simulink model "SOGI_test"  (R2016a)
settings: Solver=VariableStepAuto  StartTime=0.0  StopTime=1  RelTol=1e-3
libraries: powerlib x3, powerlib_meascontrol x2, simulink x1
settings Model: Creator=13641  LastModifiedBy=HDM

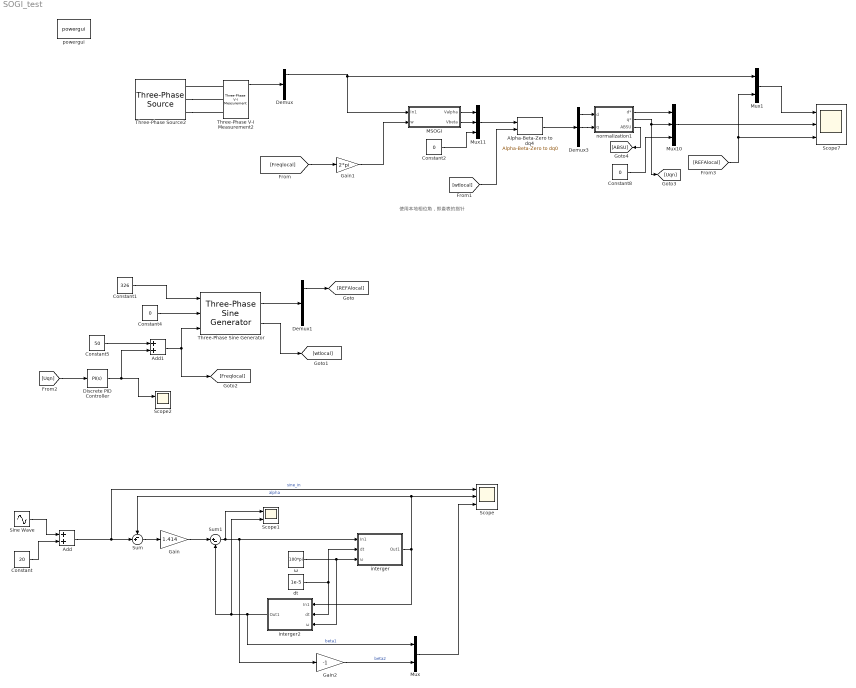
== system SOGI_test ==
  note: 使用本地相位角，即查表的指针
  Add : Sum
  Add1 : Sum
  Alpha-Beta-Zero to dq4 : powerlib_meascontrol/Transformations/Alpha-Beta-Zero to dq0  Alignment=90 degrees behind phase A axis
  Constant : Constant  Value=20
  Constant1 : Constant  Value=326
  Constant2 : Constant  Value=0
  Constant4 : Constant  Value=0
  Constant5 : Constant  Value=50
  Constant8 : Constant  Value=0
  Demux : Demux  Outputs=3
  Demux1 : Demux  Outputs=3
  Demux3 : Demux  Outputs=3
  Discrete PID Controller : simulink/Continuous/PID Controller  Controller=PI  TimeDomain=Continuous-time  SampleTime=-1  IntegratorMethod=Forward Euler  FilterMethod=Forward Euler  Form=Parallel  UseFilter=on  ControllerParametersSource=internal  P=5  I=20  D=0  N=100  InitialConditionSource=internal  InitialConditionForIntegrator=0  InitialConditionForFilter=0  ExternalReset=none  LimitOutput=off  UpperSaturationLimit=inf  LowerSaturationLimit=-inf  LinearizeAsGain=off  AntiWindupMode=none  Kb=1  TrackingMode=off  Kt=1  PParamMin=[]  PParamMax=[]  IParamMin=[]  IParamMax=[]  DParamMin=[]  DParamMax=[]  NParamMin=[]  NParamMax=[]  KbParamMin=[]  KbParamMax=[]  KtParamMin=[]  KtParamMax=[]  POutMin=[]  POutMax=[]  IOutMin=[]  IOutMax=[]  DOutMin=[]  DOutMax=[]  NOutMin=[]  NOutMax=[]  KbOutMin=[]  KbOutMax=[]  KtOutMin=[]  KtOutMax=[]  IntegratorOutMin=[]  IntegratorOutMax=[]  FilterOutMin=[]  FilterOutMax=[]  SumOutMin=[]  SumOutMax=[]  SumI1OutMin=[]  SumI1OutMax=[]  SumI2OutMin=[]  SumI2OutMax=[]  SumI3OutMin=[]  SumI3OutMax=[]  SumDOutMin=[]  SumDOutMax=[]  SaturationOutMin=[]  SaturationOutMax=[]  IntegratorContinuousStateAttributes=''  IntegratorStateMustResolveToSignalObject=off  IntegratorRTWStateStorageClass=Auto  FilterContinuousStateAttributes=''  FilterStateMustResolveToSignalObject=off  FilterRTWStateStorageClass=Auto  DifferentiatorICPrevScaledInput=0  DifferentiatorOutMin=[]  DifferentiatorOutMax=[]
  Gain : Gain  Gain=1.414
  Gain1 : Gain  Gain=2*pi
  Gain2 : Gain  Gain=-1
  MSOGI : Subsystem
  Mux : Mux  Inputs=2
  Mux1 : Mux  Inputs=2
  Mux10 : Mux  Inputs=3
  Mux11 : Mux  Inputs=3
  Scope : Scope  NumInputPorts=3
  Scope1 : Scope  NumInputPorts=2
  Scope2 : Scope  NumInputPorts=2
  Scope7 : Scope  NumInputPorts=3
  Sine Wave : Sin  Amplitude=100  Frequency=100*pi  SampleTime=1e-5
  Sum : Sum  Inputs=-+|
  Sum1 : Sum  Inputs=|+-
  Three-Phase Sine Generator : powerlib_meascontrol/Pulse & Signal Generators/Three-Phase Sine Generator  Ts=0
  Three-Phase V-I Measurement2 : powerlib/Measurements/Three-Phase V-I Measurement  VoltageMeasurement=phase-to-ground  SetLabelV=off  LabelV=Vabc  Vpu=off  VpuLL=off  CurrentMeasurement=yes  SetLabelI=off  LabelI=Iabc  Ipu=off  Pbase=100e6  Vbase=500e3  OutputType=Complex  PhasorSimulation=off  PSBequivalent=0
  Three-Phase Source2 : powerlib/Electrical Sources/Three-Phase Source  InternalConnection=Yg  VoltagePhases=off  Voltage=400  PhaseAngle=-60  Voltage_phases=[25e3 25e3 25e3]/sqrt(3)  PhaseAngles_phases=[0 -120 +120]  Frequency=50  NonIdealSource=off  SpecifyImpedance=off  Resistance=0.8929  Inductance=16.58e-3  ShortCircuitLevel=100e6  BaseVoltage=25e3  XRratio=7  BusType=swing  Pref=10e3  Qref=0  Prefabc=[10e3, 10e3, 10e3]  Qrefabc=[0, 0, 0]  Qmin=-inf  Qmax=inf
  dt : Constant  Value=1e-5
  interger : Subsystem
  interger2 : Subsystem
  normalization1 : Subsystem
  powergui : powerlib/powergui  Priority=1  SimulationMode=Discrete  SolverType=Tustin/Backward Euler (TBE)  SampleTime=0.01e-3  frequency=60  SPID=off  DisableSnubberDevices=off  DisableRonSwitches=off  DisableVfSwitches=off  SwTol=0  DisplayEquations=off  Interpol=off  ExternalGateDelay=off  methode=off  Ts=10  FunctionMessages=off  echomessages=off  HookPort=off  EnableUseOfTLC=off  x0status=blocks  frequencyindice=50  Pbase=100e6  ErrMax=1e-4  Iterations=50  UnitsV=kV  UnitsW=MW  buscounter=0  RestoreLinks=warning  ResistiveCurrentMeasurement=off  Frange=[0:2:500]  Ylog=off  Xlog=on  ShowGrid=off  save=off  variable=ZData  structure=0  ZoomFFT=off  StartTime=0.0  cycles=1  DisplayStyle=1  fundamental=60  FreqAxis=off  MaxFrequency=1000  frequencyindicesteady=1  RmsSteady=1  display=off
  ω : Constant  Value=100*pi
  wires:
  Three-Phase V-I Measurement2/1 -> Demux/1
  Constant2/1 -> Mux11/3
  MSOGI/2(Vbeta) -> Mux11/2
  MSOGI/1(Valpha) -> Mux11/1
  Mux11/1 -> Alpha-Beta-Zero to dq4/1
  Demux/1 -> MSOGI/1(In1), Mux1/1
  Demux3/2 -> normalization1/2(q)
  normalization1/1(d*) -> Mux10/1
  normalization1/2(q*) -> [Uqn], Mux10/2
  Alpha-Beta-Zero to dq4/1 -> Demux3/1
  Constant8/1 -> Mux10/3
  Mux10/1 -> Scope7/2
  [wtlocal] -> Alpha-Beta-Zero to dq4/2
  Gain1/1 -> MSOGI/2(w)
  Sum/1 -> Gain/1
  dt/1 -> interger/2(dt), interger2/2(dt)
  interger/1(Out1) -> Sum/1, Scope/2, interger2/1(In1)  "alpha"
  interger2/1(Out1) -> Mux/1, Sum1/2, Scope1/2  "beta1"
  Add/1 -> Scope/1, Sum/2  "sine_in"
  Sum1/1 -> interger/1(In1), Gain2/1, Scope1/1
  Gain/1 -> Sum1/1
  Gain2/1 -> Mux/2  "beta2"
  Mux/1 -> Scope/3
  ω/1 -> interger/3(ω), interger2/3(ω)
  Sine Wave/1 -> Add/1
  Constant/1 -> Add/2
  Constant1/1 -> Three-Phase Sine Generator/1
  Constant4/1 -> Three-Phase Sine Generator/2
  Constant5/1 -> Add1/1
  Three-Phase Sine Generator/1 -> Demux1/1
  Demux1/1 -> [REFAlocal]
  Three-Phase Sine Generator/2 -> [wtlocal]
  [Uqn] -> Discrete PID Controller/1
  Add1/1 -> [Freqlocal], Three-Phase Sine Generator/3
  [Freqlocal] -> Gain1/1
  [REFAlocal] -> Mux1/2, Scope7/3
  Discrete PID Controller/1 -> Scope2/1, Add1/2
  Demux3/1 -> normalization1/1(d)
  normalization1/3("ABSU ") -> [ABSU]
  Mux1/1 -> Scope7/1
  connections:
  Three-Phase Source2/RConn3 -- Three-Phase V-I Measurement2/LConn3
  Three-Phase Source2/RConn2 -- Three-Phase V-I Measurement2/LConn2
  Three-Phase V-I Measurement2/LConn1 -- Three-Phase Source2/RConn1

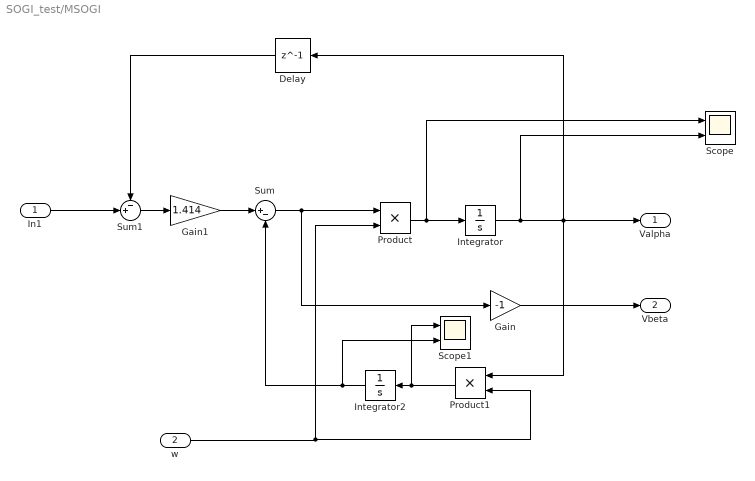
== system SOGI_test/MSOGI ==
  In1 : Inport
  w : Inport  Port=2
  Delay : Delay  DelayLength=1  InitialCondition=0  SampleTime=1e-5
  Gain : Gain  Gain=-1
  Gain1 : Gain  Gain=1.414
  Integrator : Integrator
  Integrator2 : Integrator
  Product : Product
  Product1 : Product
  Scope : Scope  NumInputPorts=2
  Scope1 : Scope  NumInputPorts=2
  Sum : Sum  Inputs=|+-
  Sum1 : Sum  Inputs=-+|
  Valpha : Outport
  Vbeta : Outport  Port=2
  wires:
  Sum/1 -> Gain/1, Product/1
  In1/1 -> Sum1/2
  Integrator2/1 -> Scope1/2, Sum/2
  Product/1 -> Scope/1, Integrator/1
  Integrator/1 -> Scope/2, Delay/1, Valpha/1, Product1/1
  Product1/1 -> Scope1/1, Integrator2/1
  w/1 -> Product/2, Product1/2
  Sum1/1 -> Gain1/1
  Gain1/1 -> Sum/1
  Gain/1 -> Vbeta/1
  Delay/1 -> Sum1/1

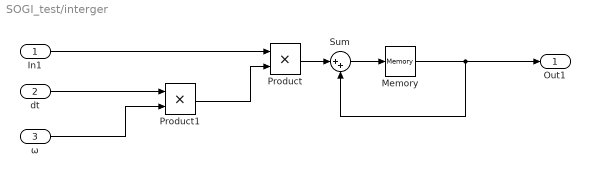
== system SOGI_test/interger ==
  In1 : Inport
  dt : Inport  Port=2
  ω : Inport  Port=3
  Memory : Memory
  Product : Product
  Product1 : Product
  Sum : Sum  Inputs=|++
  Out1 : Outport
  wires:
  Product1/1 -> Product/2
  dt/1 -> Product1/1
  Product/1 -> Sum/1
  Sum/1 -> Memory/1
  Memory/1 -> Sum/2, Out1/1
  In1/1 -> Product/1
  ω/1 -> Product1/2

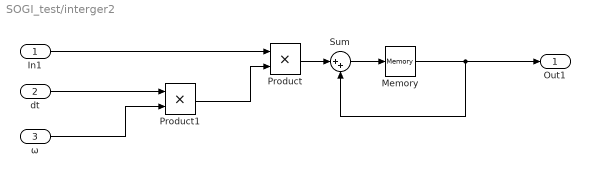
== system SOGI_test/interger2 ==
  In1 : Inport
  dt : Inport  Port=2
  ω : Inport  Port=3
  Memory : Memory
  Product : Product
  Product1 : Product
  Sum : Sum  Inputs=|++
  Out1 : Outport
  wires:
  Product1/1 -> Product/2
  dt/1 -> Product1/1
  Product/1 -> Sum/1
  Sum/1 -> Memory/1
  Memory/1 -> Sum/2, Out1/1
  In1/1 -> Product/1
  ω/1 -> Product1/2

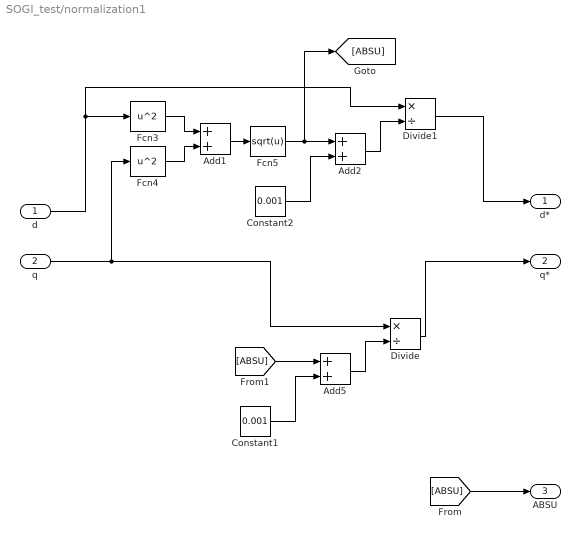
== system SOGI_test/normalization1 ==
  d : Inport
  q : Inport  Port=2
  Add1 : Sum
  Add2 : Sum
  Add5 : Sum
  Constant1 : Constant  Value=0.001
  Constant2 : Constant  Value=0.001
  Divide : Product  Inputs=*/
  Divide1 : Product  Inputs=*/
  Fcn3 : Fcn  Expr=u^2
  Fcn4 : Fcn  Expr=u^2
  Fcn5 : Fcn  Expr=sqrt(u)
  d* : Outport
  q* : Outport  Port=2
  "ABSU " : Outport  Port=3
  wires:
  Divide/1 -> q*/1
  Add5/1 -> Divide/2
  [ABSU] -> Add5/1
  q/1 -> Fcn4/1, Divide/1
  Constant1/1 -> Add5/2
  Fcn4/1 -> Add1/2
  Fcn3/1 -> Add1/1
  Divide1/1 -> d*/1
  d/1 -> Divide1/1, Fcn3/1
  Add2/1 -> Divide1/2
  Fcn5/1 -> [ABSU], Add2/1
  Add1/1 -> Fcn5/1
  Constant2/1 -> Add2/2
  [ABSU] -> "ABSU "/1
